simulink model "virtual_port_sim_prot"  (R2020b)
settings: Solver=FixedStepDiscrete  StartTime=0.0  StopTime=20  FixedStep=0.1  RelTol=1e-3
undefined symbols (not defined in the file): serial
libraries: instrumentlib x2, simulink x1
settings Model: SimulationMode=external  Creator=Mostafa  LastModifiedBy=Mostafa
settings SFSimCC: SimTargetLang=C++
settings RTWCC: Description=Simulink Desktop Real-Time  SystemTargetFile=sldrt.tlc  TemplateMakefile=sldrt.tmf  TargetLang=C++  RTWCompilerOptimization=on
settings CodeAppCC: MaxIdLength=95
settings SimulinkDesktopRealTimeCC: TargetPreCompLibLocation=C:\Program Files\Polyspace\R2020b\toolbox\sldrt\lib\win64  TargetLangStandard=C++03 (ISO)

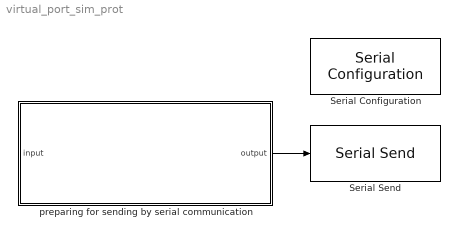
== system virtual_port_sim_prot ==
  Serial Configuration : instrumentlib/Serial Configuration  Priority=-200000  ComPortMenu=COM20  ComPort=COM20  ObjConstructor=serial('COM20');  BaudRate=9600  DataBits=8  Parity=none  StopBits=1  FlowControl=none  Timeout=10  ByteOrder=LittleEndian
  Serial Send : instrumentlib/Serial Send  ComPortMenu=COM20  ComPort=COM20  ObjConstructor=serial('COM20');  Terminator=<none>  EnableBlockingMode=on
  preparing for sending by serial communication : Subsystem
  wires:
  preparing for sending by serial communication/1(output) -> Serial Send/1

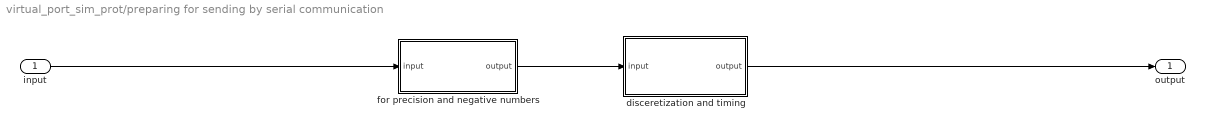
== system virtual_port_sim_prot/preparing for sending by serial communication ==
  input : Inport
  disceretization and timing : Subsystem
  for precision and negative numbers : Subsystem
  output : Outport
  wires:
  for precision and negative numbers/1(output) -> disceretization and timing/1(input)
  input/1 -> for precision and negative numbers/1(input)
  disceretization and timing/1(output) -> output/1

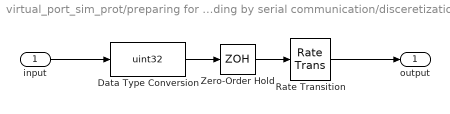
== system virtual_port_sim_prot/preparing for sending by serial communication/disceretization and timing ==
  input : Inport
  Data Type Conversion : DataTypeConversion  OutDataTypeStr=uint32
  Rate Transition : RateTransition  OutPortSampleTime=0.1
  Zero-Order Hold : ZeroOrderHold  SampleTime=0.1
  output : Outport
  wires:
  Zero-Order Hold/1 -> Rate Transition/1
  input/1 -> Data Type Conversion/1
  Data Type Conversion/1 -> Zero-Order Hold/1
  Rate Transition/1 -> output/1

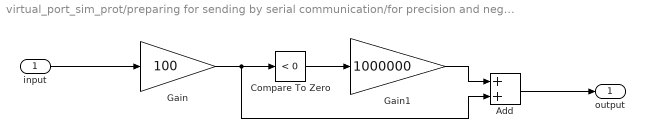
== system virtual_port_sim_prot/preparing for sending by serial communication/for precision and negative numbers ==
  input : Inport
  Add : Sum
  Compare To Zero : simulink/Logic and Bit Operations/Compare To Zero  relop=<  OutDataTypeStr=boolean
  Gain : Gain  Gain=100
  Gain1 : Gain  Gain=1000000  ParamDataTypeStr=double  OutDataTypeStr=double
  output : Outport
  wires:
  Compare To Zero/1 -> Gain1/1
  Add/1 -> output/1
  Gain1/1 -> Add/1
  Gain/1 -> Add/2, Compare To Zero/1
  input/1 -> Gain/1
